simulink model "sim_task_2"  (R2024a)
settings: Solver=FixedStepAuto  StartTime=0.0  StopTime=10.0  FixedStep=1e-3  RelTol=1e-3
settings Model: Creator=alexe  LastModifiedBy=alexe

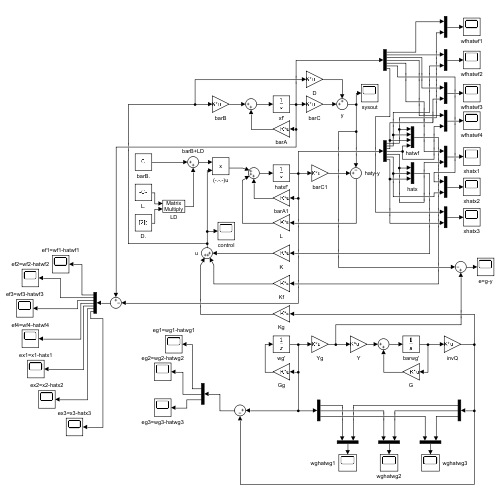
[thumbnail: Simulink's stored preview of the top-level diagram]
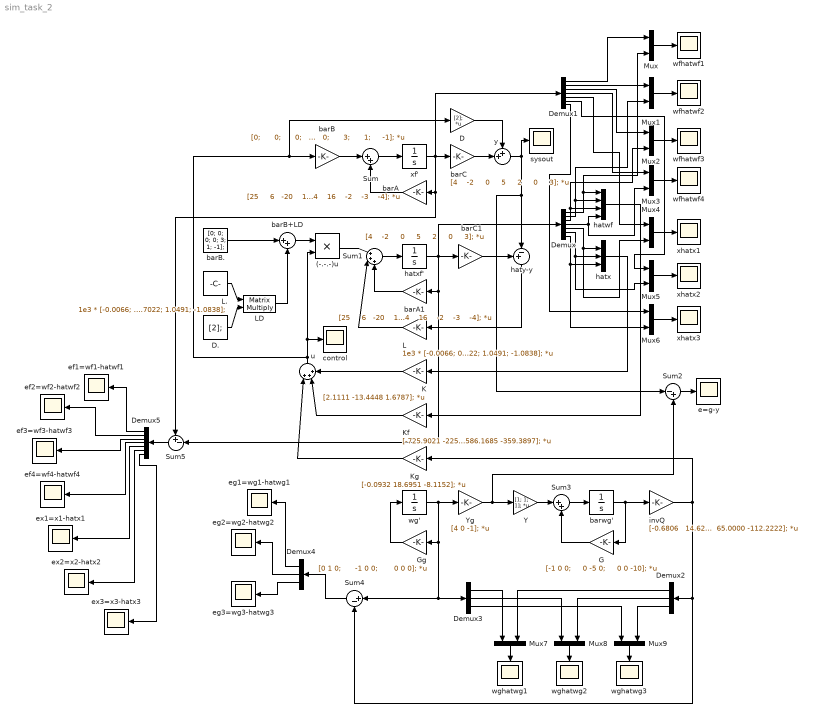
== system sim_task_2 ==
  (-.-.-)u : Product
  D : Gain  Gain=[2];  Multiplication=Matrix(K*u)
  D. : Constant  Value=[2];  VectorParams1D=off
  Demux : Demux  Outputs=7
  Demux1 : Demux  Outputs=7
  Demux2 : Demux  Outputs=3
  Demux3 : Demux  Outputs=3
  Demux4 : Demux  Outputs=3
  Demux5 : Demux  Outputs=7
  G : Gain  Gain=|  Multiplication=Matrix(K*u)
      | [-1 0 0;
      |     0 -5 0;
      |     0 0 -10];
  Gg : Gain  Gain=|  Multiplication=Matrix(K*u)
      | [0 1 0;
      |      -1 0 0;
      |       0 0 0];
  K : Gain  Gain=[2.1111 -13.4448 1.6787];  Multiplication=Matrix(K*u)
  Kf : Gain  Gain=[-725.9021 -225.1491 586.1685 -359.3897];  Multiplication=Matrix(K*u)
  Kg : Gain  Gain=[-0.0932 18.6951 -8.1152];  Multiplication=Matrix(K*u)
  L : Gain  Gain=1e3 * [-0.0066; 0.0219; -0.0143; -0.0229; 1.7022; 1.0491; -1.0838];  Multiplication=Matrix(K*u)
  L. : Constant  Value=1e3 * [-0.0066; 0.0219; -0.0143; -0.0229; 1.7022; 1.0491; -1.0838];  VectorParams1D=off
  LD : Product  Multiplication=Matrix(*)
  Mux{,1..9} (10 alike) : Mux  Inputs=2
  Sum : Sum  Inputs=|++
  Sum1 : Sum  Inputs=|+++
  Sum2 : Sum  Inputs=|-+
  Sum3 : Sum  Inputs=|++
  Sum4 : Sum  Inputs=|+-
  Sum5 : Sum  Inputs=+-|
  Y : Gain  Gain=[1; 1; 1];  Multiplication=Matrix(K*u)
  Yg : Gain  Gain=[4 0 -1];  Multiplication=Matrix(K*u)
  barA : Gain  Gain="[25     6   -20    11     0     0     0; 14     3   -10     4     0     0     0; 40    11   -31    17     0     0     0; 6     4    -4     3     0     0     0; -12    -2     8    -7     5     2     7; 0     0     0     0     2     1     2; 32     8   -24    16    -2    -3    -4];"  Multiplication=Matrix(K*u)
  barA1 : Gain  Gain="[25     6   -20    11     0     0     0; 14     3   -10     4     0     0     0; 40    11   -31    17     0     0     0; 6     4    -4     3     0     0     0; -12    -2     8    -7     5     2     7; 0     0     0     0     2     1     2; 32     8   -24    16    -2    -3    -4];"  Multiplication=Matrix(K*u)
  barB : Gain  Gain=|  Multiplication=Matrix(K*u)
      | [0;
      |      0;
      |      0;
      |      0;
      |      3;
      |      1;
      |     -1];
  barB+LD : Sum  Inputs=|++
  barB. : Constant  Value=|  VectorParams1D=off
      | [0;
      |      0;
      |      0;
      |      0;
      |      3;
      |      1;
      |     -1];
  barC : Gain  Gain="[4    -2     0     5     2     0     3];"  Multiplication=Matrix(K*u)
  barC1 : Gain  Gain="[4    -2     0     5     2     0     3];"  Multiplication=Matrix(K*u)
  barwg' : Integrator  InitialCondition=[0;0;0];
  control : Scope
  e=g-y : Scope
  ef1=wf1-hatwf1 : Scope
  ef2=wf2-hatwf2 : Scope
  ef3=wf3-hatwf3 : Scope
  ef4=wf4-hatwf4 : Scope
  eg1=wg1-hatwg1 : Scope
  eg2=wg2-hatwg2 : Scope
  eg3=wg3-hatwg3 : Scope
  ex1=x1-hatx1 : Scope
  ex2=x2-hatx2 : Scope
  ex3=x3-hatx3 : Scope
  hatwf : Mux
  hatx : Mux  Inputs=3
  hatxf' : Integrator  InitialCondition=[0;0;0;0;0;0;0];
  haty-y : Sum  Inputs=+-|
  invQ : Gain  Gain=|  Multiplication=Matrix(K*u)
      | [-0.6806   14.6250  -22.4444;
      |     0.2083  -17.8750   33.6667;
      |    -2.7778   65.0000 -112.2222];
  sysout : Scope
  u : Sum  Inputs=|+++
  wfhatwf{1..4} (4 alike) : Scope
  wg' : Integrator  InitialCondition=[0;1;1];
  wghatwg1 : Scope
  wghatwg2 : Scope
  wghatwg3 : Scope
  xf' : Integrator  InitialCondition=[1;1;1;1;0;0;0];
  xhatx1 : Scope
  xhatx2 : Scope
  xhatx3 : Scope
  y : Sum  Inputs=++|
  wires:
  barB/1 -> Sum/1
  Sum/1 -> xf'/1
  barA/1 -> Sum/2
  xf'/1 -> Demux1/1, Sum5/1, barA/1, barC/1
  barC/1 -> y/2
  D/1 -> y/1
  hatxf'/1 -> Demux/1, barC1/1, Sum5/2, barA1/1
  L./1 -> LD/1
  D./1 -> LD/2
  LD/1 -> barB+LD/2
  barB./1 -> barB+LD/1
  barB+LD/1 -> (-.-.-)u/1
  Sum1/1 -> hatxf'/1
  barA1/1 -> Sum1/3
  (-.-.-)u/1 -> Sum1/1
  y/1 -> sysout/1, Sum2/1, haty-y/2
  barC1/1 -> haty-y/1
  haty-y/1 -> L/1
  L/1 -> Sum1/2
  Demux/1 -> hatwf/1, Mux/2
  Demux/2 -> hatwf/2, Mux1/2
  Demux/3 -> Mux2/2, hatwf/3
  Demux/4 -> hatwf/4, Mux3/2
  Demux/5 -> Mux4/2, hatx/1
  Demux/6 -> Mux5/2, hatx/2
  Demux/7 -> Mux6/2, hatx/3
  hatx/1 -> K/1
  hatwf/1 -> Kf/1
  u/1 -> control/1, (-.-.-)u/2, D/1, barB/1
  K/1 -> u/3
  Kf/1 -> u/2
  Kg/1 -> u/1
  Demux1/5 -> Mux4/1
  Demux1/6 -> Mux5/1
  Demux1/7 -> Mux6/1
  Gg/1 -> wg'/1
  wg'/1 -> Yg/1, Sum4/1, Demux3/1, Gg/1
  Yg/1 -> Sum2/2, Y/1
  barwg'/1 -> invQ/1, G/1
  Y/1 -> Sum3/1
  Sum3/1 -> barwg'/1
  G/1 -> Sum3/2
  invQ/1 -> Sum4/2, Demux2/1, Kg/1
  Mux/1 -> wfhatwf1/1
  Demux1/1 -> Mux/1
  Demux1/2 -> Mux1/1
  Demux1/3 -> Mux2/1
  Demux1/4 -> Mux3/1
  Mux1/1 -> wfhatwf2/1
  Mux2/1 -> wfhatwf3/1
  Mux3/1 -> wfhatwf4/1
  Mux6/1 -> xhatx3/1
  Mux5/1 -> xhatx2/1
  Mux4/1 -> xhatx1/1
  Demux3/1 -> Mux7/1
  Demux2/1 -> Mux7/2
  Demux3/2 -> Mux8/1
  Demux2/2 -> Mux8/2
  Demux3/3 -> Mux9/1
  Demux2/3 -> Mux9/2
  Mux7/1 -> wghatwg1/1
  Mux8/1 -> wghatwg2/1
  Mux9/1 -> wghatwg3/1
  Sum2/1 -> e=g-y/1
  Sum4/1 -> Demux4/1
  Demux4/1 -> eg1=wg1-hatwg1/1
  Demux4/2 -> eg2=wg2-hatwg2/1
  Demux4/3 -> eg3=wg3-hatwg3/1
  Sum5/1 -> Demux5/1
  Demux5/1 -> ef1=wf1-hatwf1/1
  Demux5/2 -> ef2=wf2-hatwf2/1
  Demux5/3 -> ef3=wf3-hatwf3/1
  Demux5/4 -> ef4=wf4-hatwf4/1
  Demux5/5 -> ex1=x1-hatx1/1
  Demux5/6 -> ex2=x2-hatx2/1
  Demux5/7 -> ex3=x3-hatx3/1
